simulink model "imageProcessing_th"  (R2018a)
settings: Solver=FixedStepDiscrete  StartTime=0.0  StopTime=0  RelTol=1e-3
StopFcn:
  | imshow(image.signals.values)
undefined symbols (not defined in the file or in its folder): Rec, SDTV
libraries: visionconversions x1, visionsources x1, ImageProcessing_cl x1
settings Model: Creator=mcobb  LastModifiedBy=mcobb

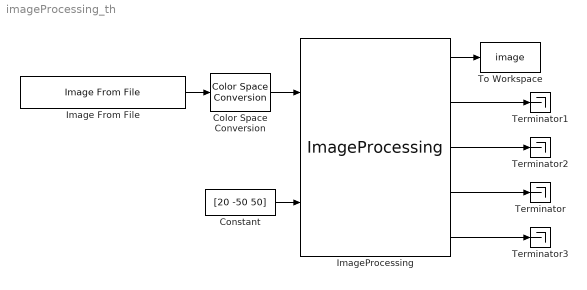
== system imageProcessing_th ==
  Color Space Conversion : visionconversions/Color Space  Conversion  conversion=Obsolete  conversionActive=R'G'B' to intensity  wp_str=D65  rec=Rec. 601 (SDTV)  sys=1125/60/2:1  imagePorts=One multidimensional signal
      settings: SourceProductName=Computer Vision System Toolbox
  Constant : Constant  Value=[20 -50 50]
  Image From File : visionsources/Image From File  Tag=vipblks_nd  FileName=C:\Users\mcobb\Google Drive\speedgoatTest\test4\testImage.PNG  imagePorts=One multidimensional signal  Ts=inf  ImageDataType=Inherit from input image  Signed=on  WordLength=16  sdImageDataType=uint(8)  FractionLengthMode=User-defined  FractionLength=15  OutPortLabels=R|G|B
      settings: SourceProductName=Computer Vision System Toolbox
  ImageProcessing : ImageProcessing_cl/ImageProcessing  ROIPositionHoldEnable=on  ROIPositionHoldCoordinates=[374 560]  ROIDimVec_px=[120 50]  ROIHalfDimVec_px=[15 45]  ROISplitDims_px=[1 15 ; 1 90 ; 16 14 ; 1 90]  DotOrientation=Vertical  OverlayOutput=on  ImageDimensions=[765 998]  CrosshairPixelWidth_px=1  camPositionVec_cm=[20 -50 50]  camFOVVec_deg=[30 30]
  Terminator{,1..3} (4 alike) : Terminator
  To Workspace : ToWorkspace  VariableName=image  SaveFormat=Structure With Time  SampleTime=-1
  wires:
  Image From File/1 -> Color Space Conversion/1
  Color Space Conversion/1 -> ImageProcessing/1
  Constant/1 -> ImageProcessing/2
  ImageProcessing/2 -> Terminator1/1
  ImageProcessing/3 -> Terminator2/1
  ImageProcessing/5 -> Terminator3/1
  ImageProcessing/4 -> Terminator/1
  ImageProcessing/1 -> To Workspace/1
